simulink model "ScriptDemo"  (R2022b)
settings: configuration reference "TmVcThermal_Configuration_sub" (kept outside this file)
undefined symbols (not defined in the file): aaaa, bbbb, cTmComprCtrl_D_u8HvacFlowTable_db, cTmComprCtrl_D_u8HvacFlowTable_sw, cTmComprCtrl_n_i16ChillCmpIMax, cTmComprCtrl_n_i16ChillCmpIMin, cTmComprCtrl_n_i16ChillCmpIMin666, cTmComprCtrl_n_i16ChillCmpPMax, cTmComprCtrl_n_i16ChillCmpPMin, cTmComprCtrl_n_i16CmpChillCoolRpmKiMax, cTmComprCtrl_n_i16CmpChillCoolRpmKiMin, cTmComprCtrl_n_i16CmpChillCoolRpmKpMax, cTmComprCtrl_n_i16CmpChillCoolRpmKpMin, cTmComprCtrl_n_i16CmpCoolRpmKiMax, cTmComprCtrl_n_i16CmpCoolRpmKiMin, cTmComprCtrl_n_i16CmpCoolRpmKpMax, cTmComprCtrl_n_i16CmpCoolRpmKpMin, cTmComprCtrl_n_i16SM4CmpHeatKiMax, cTmComprCtrl_n_i16SM4CmpHeatKiMin, cTmComprCtrl_n_i16SM4CmpHeatKpMax, cTmComprCtrl_n_i16SM4CmpHeatKpMin, cTmComprCtrl_n_i16SM5CmpHeatKiMax, cTmComprCtrl_n_i16SM5CmpHeatKiMin, cTmComprCtrl_n_i16SM5CmpHeatKpMax, cTmComprCtrl_n_i16SM5CmpHeatKpMin, cTmComprCtrl_n_i16SM6CmpHeatKiMax, cTmComprCtrl_n_i16SM6CmpHeatKiMin, cTmComprCtrl_n_i16SM6CmpHeatKpMax, cTmComprCtrl_n_i16SM6CmpHeatKpMin, cTmComprCtrl_n_u16CmpMaxSpdFanFltLimt, cTmComprCtrl_n_u16CmpMaxSpdLoSidePFltLimt, cTmComprCtrl_n_u16CmpMaxSpdSensorFltLimt, cTmComprCtrl_n_u16CompMinRpm, cTmComprCtrl_n_u16CompRpmIncThres, cTmComprCtrl_t_u16BattCooltFFPeriod, cTmComprCtrl_t_u16BattCooltPIPeriod, cTmComprCtrl_t_u16CmpCoolFFPeriod, cTmComprCtrl_t_u16CmpCoolPIPeriod, cTmComprCtrl_t_u16CoolCmpChillFFPeriod, cTmComprCtrl_t_u16CoolCmpChillPIPeriod, cTmComprCtrl_t_u16SM4CmpHeatFFPeriod, cTmComprCtrl_t_u16SM4CmpHeatPIPeriod, cTmComprCtrl_t_u16SM5CmpHeatFFPeriod, cTmComprCtrl_t_u16SM5CmpHeatPIPeriod, cTmComprCtrl_t_u16SM6CmpHeatFFPeriod, cTmComprCtrl_t_u16SM6CmpHeatPIPeriod, cTmComprCtrl_Te_EvapClearInteg, cTmComprCtrl_Te_i16HpReqTempSaturoffset, cTmComprCtrl_Te_i16SatLpReplaceDiff, cTmComprCtrl_Te_i16SM3BatDiffStartEvapDecOffset, cTmComprCtrl_Te_i16SM3EvapLo, cTmComprCtrl_Te_i16SM3TBatDiffEntEvapDecOffset, cTmComprCtrl_Te_i16SM3TBatDiffEntEvapDecOffsetQuit, cTmComprCtrl_Te_s32ErrCmpChillPIContinueCoolH, cTmComprCtrl_Te_s32ErrCmpChillPIContinueCoolL, cTmComprCtrl_Te_s32ErrCmpPIContinueChillH, cTmComprCtrl_Te_s32ErrCmpPIContinueChillL, cTmComprCtrl_Te_s32ErrCmpPIContinueCoolH, cTmComprCtrl_Te_s32ErrCmpPIContinueCoolL, cTmComprCtrl_Te_s32ErrCmpPIContinueHeatH ... (+398)
libraries: simulink x782, PCMULib x640, simulink_need_slupdate x4
(part 21 of 41)

== system ScriptDemo/Create/createMerge/After/SM4/ID26297_SM4FF ==
  sTmComprCtrl_D_u8HvacFlowLevel : Inport  OutDataTypeStr=uint8
  sTmSigProces_Te_s32TempInlet : Inport  Port=2
  sTmSigProces_Te_s32HeatrAirTReqRamp : Inport  Port=3
  sTmSigProces_Te_s32TAmb : Inport  Port=4  OutDataTypeStr=single
  Enable : EnablePort
  1-D Lookup Table : Lookup_n-D  NumberOfTableDimensions=1  BreakpointsForDimension1=tTmComprCtrl_fac_s32FFSM4CompHeatAmbFactor_X  BreakpointsForDimension1DataTypeStr=Inherit: Inherit from 'Breakpoint data'  Table=tTmComprCtrl_fac_s32FFSM4CompHeatAmbFactor  TableDataTypeStr=Inherit: Inherit from 'Table data'  ExtrapMethod=Clip  InternalRulePriority=Speed  OutDataTypeStr=Inherit: Inherit via back propagation  RndMeth=Simplest  InputSameDT=off
  Flow2Rpm : Subsystem  mask{BlwHeatLevel_db=cTmComprCtrl_D_u8HvacFlowTable_db, BlwHeatLevel_sw=cTmComprCtrl_D_u8HvacFlowTable_sw, FFBlw1=mTmComprCtrl_n_u16FFSM4CompHeatRpm_Flow1, FFBlw1_Y=mTmComprCtrl_n_u16FFSM4CompHeatRpm_Flow1_Y, FFBlw1_X=mTmComprCtrl_n_u16FFSM4CompHeatRpm_Flow1_X, FFBlw3=mTmComprCtrl_n_u16FFSM4CompHeatRpm_Flow3, FFBlw3_Y=mTmComprCtrl_n_u16FFSM4CompHeatRpm_Flow3_Y, FFBlw3_X=mTmComprCtrl_n_u16FFSM4CompHeatRpm_Flow3_X, FFBlw5=mTmComprCtrl_n_u16FFSM4CompHeatRpm_Flow5, FFBlw5_Y=mTmComprCtrl_n_u16FFSM4CompHeatRpm_Flow5_Y, FFBlw5_X=mTmComprCtrl_n_u16FFSM4CompHeatRpm_Flow5_X, FFBlw7=mTmComprCtrl_n_u16FFSM4CompHeatRpm_Flow7, FFBlw7_Y=mTmComprCtrl_n_u16FFSM4CompHeatRpm_Flow7_Y, FFBlw7_X=mTmComprCtrl_n_u16FFSM4CompHeatRpm_Flow7_X, FFBlw9=mTmComprCtrl_n_u16FFSM4CompHeatRpm_Flow9, FFBlw9_Y=mTmComprCtrl_n_u16FFSM4CompHeatRpm_Flow9_Y, FFBlw9_X=mTmComprCtrl_n_u16FFSM4CompHeatRpm_Flow9_X}
      mask DialogControl ParameterGroupVar Prompt: 参数
  Product : Product  OutDataTypeStr=uint16
  SM4FF : Outport
  wires:
  sTmComprCtrl_D_u8HvacFlowLevel/1 -> Flow2Rpm/1(md_u8Blw)
  sTmSigProces_Te_s32TempInlet/1 -> Flow2Rpm/2(breakpoint1)
  sTmSigProces_Te_s32HeatrAirTReqRamp/1 -> Flow2Rpm/3(breakpoint2)
  [sTmSigProces_Te_s32TAmb] -> 1-D Lookup Table/1
  1-D Lookup Table/1 -> Product/2  "rTmComprCtrl_fac_s32FFSM4CompHeatAmbFactor"
  Flow2Rpm/1(Flow2Rpm) -> Product/1  "rTmComprCtrl_n_u16FFSM4CompHeatRpm"
  Product/1 -> SM4FF/1
  sTmSigProces_Te_s32TAmb/1 -> [sTmSigProces_Te_s32TAmb]

== system ScriptDemo/Create/createMerge/After/SM4/SM24FFEnable ==
  xTmComprCtrl_B_CompOnReqCompOn : Inport  OutDataTypeStr=boolean
  Compare To Constant2 : simulink/Logic and Bit Operations/Compare To Constant  relop===  const=0  OutDataTypeStr=boolean
  Compare To Constant3 : simulink/Logic and Bit Operations/Compare To Constant  relop===  const=1  OutDataTypeStr=boolean
  Logical Operator3 : Logic  AllPortsSameDT=off  OutDataTypeStr=boolean
  PeriodTrig : Subsystem  mask{CounterLim=cTmComprCtrl_t_u16SM4CmpHeatFFPeriod}
      mask DialogControl ParameterGroupVar Prompt: 参数
  Unit Delay : UnitDelay  SampleTime=-1  HasFrameUpgradeWarning=on
  SM4FFEnable_B_SM4FFEnable : Outport  OutDataTypeStr=boolean
  wires:
  Unit Delay/1 -> Compare To Constant2/1
  [xTmComprCtrl_B_CompOnReqCompOn] -> Compare To Constant3/1, Unit Delay/1
  Compare To Constant2/1 -> Logical Operator3/1
  Logical Operator3/1 -> PeriodTrig/1(Counter_Reset)
  Compare To Constant3/1 -> Logical Operator3/2
  xTmComprCtrl_B_CompOnReqCompOn/1 -> [xTmComprCtrl_B_CompOnReqCompOn]
  PeriodTrig/1(Counter_Trig) -> SM4FFEnable_B_SM4FFEnable/1

== system ScriptDemo/Create/createMerge/After/SM4/SM4_Ki ==
  sTmComprCtrl_D_u8HvacFlowLevel : Inport  OutDataTypeStr=uint8
  sTmSigProces_Te_s32TAmb : Inport  Port=2
  rTmComprCtrl_Te_s32TempError : Inport  Port=3
  Flow2Rpm : Subsystem  mask{BlwHeatLevel_db=cTmComprCtrl_D_u8HvacFlowTable_db, BlwHeatLevel_sw=cTmComprCtrl_D_u8HvacFlowTable_sw, FFBlw1=mTmComprCtrl_n_u16KiSM4CompHeatRpm_Flow1, FFBlw1_Y=mTmComprCtrl_n_u16KiSM4CompHeatRpm_Flow1_Y, FFBlw1_X=mTmComprCtrl_n_u16KiSM4CompHeatRpm_Flow1_X, FFBlw3=mTmComprCtrl_n_u16KiSM4CompHeatRpm_Flow3, FFBlw3_Y=mTmComprCtrl_n_u16KiSM4CompHeatRpm_Flow3_Y, FFBlw3_X=mTmComprCtrl_n_u16KiSM4CompHeatRpm_Flow3_X, FFBlw5=mTmComprCtrl_n_u16KiSM4CompHeatRpm_Flow5, FFBlw5_Y=mTmComprCtrl_n_u16KiSM4CompHeatRpm_Flow5_Y, FFBlw5_X=mTmComprCtrl_n_u16KiSM4CompHeatRpm_Flow5_X, FFBlw7=mTmComprCtrl_n_u16KiSM4CompHeatRpm_Flow7, FFBlw7_Y=mTmComprCtrl_n_u16KiSM4CompHeatRpm_Flow7_Y, FFBlw7_X=mTmComprCtrl_n_u16KiSM4CompHeatRpm_Flow7_X, FFBlw9=mTmComprCtrl_n_u16KiSM4CompHeatRpm_Flow9, FFBlw9_Y=mTmComprCtrl_n_u16KiSM4CompHeatRpm_Flow9_Y, FFBlw9_X=mTmComprCtrl_n_u16KiSM4CompHeatRpm_Flow9_X}
      mask DialogControl ParameterGroupVar Prompt: 参数
  SM4Ki : Outport
  wires:
  Flow2Rpm/1(Flow2Rpm) -> SM4Ki/1  "mask"
  sTmComprCtrl_D_u8HvacFlowLevel/1 -> Flow2Rpm/1(md_u8Blw)
  sTmSigProces_Te_s32TAmb/1 -> Flow2Rpm/2(breakpoint1)
  rTmComprCtrl_Te_s32TempError/1 -> Flow2Rpm/3(breakpoint2)

== system ScriptDemo/Create/createMerge/After/SM4/SM4_Kp ==
  sTmComprCtrl_D_u8HvacFlowLevel : Inport  OutDataTypeStr=uint8
  sTmSigProces_Te_s32TAmb : Inport  Port=2
  rTmComprCtrl_Te_s32TempError : Inport  Port=3
  Flow2Rpm : Subsystem  mask{BlwHeatLevel_db=cTmComprCtrl_D_u8HvacFlowTable_db, BlwHeatLevel_sw=cTmComprCtrl_D_u8HvacFlowTable_sw, FFBlw1=mTmComprCtrl_n_u16KpSM4CompHeatRpm_Flow1, FFBlw1_Y=mTmComprCtrl_n_u16KpSM4CompHeatRpm_Flow1_Y, FFBlw1_X=mTmComprCtrl_n_u16KpSM4CompHeatRpm_Flow1_X, FFBlw3=mTmComprCtrl_n_u16KpSM4CompHeatRpm_Flow3, FFBlw3_Y=mTmComprCtrl_n_u16KpSM4CompHeatRpm_Flow3_Y, FFBlw3_X=mTmComprCtrl_n_u16KpSM4CompHeatRpm_Flow3_X, FFBlw5=mTmComprCtrl_n_u16KpSM4CompHeatRpm_Flow5, FFBlw5_Y=mTmComprCtrl_n_u16KpSM4CompHeatRpm_Flow5_Y, FFBlw5_X=mTmComprCtrl_n_u16KpSM4CompHeatRpm_Flow5_X, FFBlw7=mTmComprCtrl_n_u16KpSM4CompHeatRpm_Flow7, FFBlw7_Y=mTmComprCtrl_n_u16KpSM4CompHeatRpm_Flow7_Y, FFBlw7_X=mTmComprCtrl_n_u16KpSM4CompHeatRpm_Flow7_X, FFBlw9=mTmComprCtrl_n_u16KpSM4CompHeatRpm_Flow9, FFBlw9_Y=mTmComprCtrl_n_u16KpSM4CompHeatRpm_Flow9_Y, FFBlw9_X=mTmComprCtrl_n_u16KpSM4CompHeatRpm_Flow9_X}
      mask DialogControl ParameterGroupVar Prompt: 参数
  SM4Kp : Outport
  wires:
  Flow2Rpm/1(Flow2Rpm) -> SM4Kp/1  "mask"
  sTmComprCtrl_D_u8HvacFlowLevel/1 -> Flow2Rpm/1(md_u8Blw)
  sTmSigProces_Te_s32TAmb/1 -> Flow2Rpm/2(breakpoint1)
  rTmComprCtrl_Te_s32TempError/1 -> Flow2Rpm/3(breakpoint2)

== system ScriptDemo/Create/createMerge/After/SM5/ID26291_SM5FF ==
  note: SM5前馈值
  note: SM5前馈值修正系数
  sTmComprCtrl_D_u8HvacFlowLevel : Inport  OutDataTypeStr=uint8
  sTmSigProces_Te_s32TempInlet : Inport  Port=2
  sTmSigProces_Te_s32HeatrAirTReqRamp : Inport  Port=3
  sTmSigProces_Te_s32SatLp : Inport  Port=4
  Enable : EnablePort
  2-D Lookup Table5 : Lookup_n-D  NumberOfTableDimensions=1  BreakpointsForDimension1=tTmComprCtrl_fac_s32FFSM5CompHeatBattCooltTFactor_X  BreakpointsForDimension2=mTmComprCtrl_n_u16FFSM5CompHeatRpmOffset_X  BreakpointsForDimension1DataTypeStr=Inherit: Inherit from 'Breakpoint data'  BreakpointsForDimension2DataTypeStr=Inherit: Inherit from 'Breakpoint data'  Table=tTmComprCtrl_fac_s32FFSM5CompHeatBattCooltTFactor  TableDataTypeStr=Inherit: Inherit from 'Table data'  ExtrapMethod=Clip  InternalRulePriority=Speed  OutDataTypeStr=Inherit: Inherit via back propagation  RndMeth=Simplest  InputSameDT=off
  Data Type Conversion : DataTypeConversion  OutDataTypeStr=uint16  SaturateOnIntegerOverflow=off  RndMeth=Floor
  Flow2Rpm : Subsystem  mask{BlwHeatLevel_db=cTmComprCtrl_D_u8HvacFlowTable_db, BlwHeatLevel_sw=cTmComprCtrl_D_u8HvacFlowTable_sw, FFBlw1=mTmComprCtrl_n_u16FFSM5CompHeatRpm_Flow1, FFBlw1_Y=mTmComprCtrl_n_u16FFSM5CompHeatRpm_Flow1_Y, FFBlw1_X=mTmComprCtrl_n_u16FFSM5CompHeatRpm_Flow1_X, FFBlw3=mTmComprCtrl_n_u16FFSM5CompHeatRpm_Flow3, FFBlw3_Y=mTmComprCtrl_n_u16FFSM5CompHeatRpm_Flow3_Y, FFBlw3_X=mTmComprCtrl_n_u16FFSM5CompHeatRpm_Flow3_X, FFBlw5=mTmComprCtrl_n_u16FFSM5CompHeatRpm_Flow5, FFBlw5_Y=mTmComprCtrl_n_u16FFSM5CompHeatRpm_Flow5_Y, FFBlw5_X=mTmComprCtrl_n_u16FFSM5CompHeatRpm_Flow5_X, FFBlw7=mTmComprCtrl_n_u16FFSM5CompHeatRpm_Flow7, FFBlw7_Y=mTmComprCtrl_n_u16FFSM5CompHeatRpm_Flow7_Y, FFBlw7_X=mTmComprCtrl_n_u16FFSM5CompHeatRpm_Flow7_X, FFBlw9=mTmComprCtrl_n_u16FFSM5CompHeatRpm_Flow9, FFBlw9_Y=mTmComprCtrl_n_u16FFSM5CompHeatRpm_Flow9_Y, FFBlw9_X=mTmComprCtrl_n_u16FFSM5CompHeatRpm_Flow9_X}
      mask DialogControl ParameterGroupVar Prompt: 参数
  Product : Product  OutDataTypeStr=uint16
  SM5FF : Outport
  wires:
  sTmSigProces_Te_s32SatLp/1 -> 2-D Lookup Table5/1
  2-D Lookup Table5/1 -> Product/2  "rTmComprCtrl_fac_s32FFSM5CompHeatBattCooltTFactor"
  Product/1 -> SM5FF/1
  sTmComprCtrl_D_u8HvacFlowLevel/1 -> Flow2Rpm/1(md_u8Blw)
  sTmSigProces_Te_s32TempInlet/1 -> Flow2Rpm/2(breakpoint1)
  sTmSigProces_Te_s32HeatrAirTReqRamp/1 -> Flow2Rpm/3(breakpoint2)
  Flow2Rpm/1(Flow2Rpm) -> Data Type Conversion/1
  Data Type Conversion/1 -> Product/1  "rTmComprCtrl_n_u16FFSM5CompHeatRpm"

== system ScriptDemo/Create/createMerge/After/SM5/ID26293_SM5Error ==
  note: 未实现
      | 暖风芯体背风温度目标值∈[30, 60] ℃ 。
  note: 无PTC补热
  note: PTC 补热模式
  sTmSigProces_Te_s32SatHp : Inport
  yTmHvchCtrl_B_HpcPtcEnad : Inport  Port=2
  sTmSigProces_Te_s32HeatrAirTReqRamp : Inport  Port=3
  sTmSigProces_Te_s32HvacHexAirTFilter : Inport  Port=4
  Add2 : Sum
  Constant5 : Constant  Value=cTmComprCtrl_Te_i16HpReqTempSaturoffset
  NegAndPosCheck 4 : Subsystem  AncestorBlock=CustomLib/TempNegAndPosCheck
  NegAndPosCheck 5 : Subsystem  AncestorBlock=CustomLib/TempNegAndPosCheck
  Saturation3 : Saturate  UpperLimit=70  LowerLimit=15
  Switch2 : Switch  Criteria=u2 ~= 0  SaturateOnIntegerOverflow=off  InputSameDT=off
  Terminator : Terminator
  Terminator1 : Terminator
  Unary Minus : UnaryMinus
  rTmComprCtrl_Te_s32TempError : Outport
  wires:
  sTmSigProces_Te_s32SatHp/1 -> NegAndPosCheck 4/2(Acture)
  NegAndPosCheck 5/1(Dvt) -> Switch2/3
  sTmSigProces_Te_s32HeatrAirTReqRamp/1 -> Saturation3/1
  Switch2/1 -> Unary Minus/1
  NegAndPosCheck 5/2(Dvt_PosFlag) -> Terminator/1
  NegAndPosCheck 4/1(Dvt) -> Switch2/1
  Constant5/1 -> Add2/1
  NegAndPosCheck 4/2(Dvt_PosFlag) -> Terminator1/1
  sTmSigProces_Te_s32HvacHexAirTFilter/1 -> NegAndPosCheck 5/2(Acture)
  yTmHvchCtrl_B_HpcPtcEnad/1 -> Switch2/2
  Saturation3/1 -> NegAndPosCheck 5/1(SetPoint), Add2/2
  Add2/1 -> NegAndPosCheck 4/1(SetPoint)
  Unary Minus/1 -> rTmComprCtrl_Te_s32TempError/1

== system ScriptDemo/Create/createMerge/After/SM5/SM5FFEnable ==
  xTmComprCtrl_B_CompOnReqCompOn : Inport  OutDataTypeStr=boolean
  Compare To Constant2 : simulink/Logic and Bit Operations/Compare To Constant  relop===  const=0  OutDataTypeStr=boolean
  Compare To Constant3 : simulink/Logic and Bit Operations/Compare To Constant  relop===  const=1  OutDataTypeStr=boolean
  Logical Operator3 : Logic  AllPortsSameDT=off  OutDataTypeStr=boolean
  PeriodTrig : Subsystem  mask{CounterLim=cTmComprCtrl_t_u16SM5CmpHeatFFPeriod}
      mask DialogControl ParameterGroupVar Prompt: 参数
  Unit Delay : UnitDelay  SampleTime=-1  HasFrameUpgradeWarning=on
  SM5FFEnable_B_SM5FFEnable : Outport  OutDataTypeStr=boolean
  wires:
  Unit Delay/1 -> Compare To Constant2/1
  [xTmComprCtrl_B_CompOnReqCompOn] -> Compare To Constant3/1, Unit Delay/1
  Compare To Constant2/1 -> Logical Operator3/1
  Logical Operator3/1 -> PeriodTrig/1(Counter_Reset)
  Compare To Constant3/1 -> Logical Operator3/2
  xTmComprCtrl_B_CompOnReqCompOn/1 -> [xTmComprCtrl_B_CompOnReqCompOn]
  PeriodTrig/1(Counter_Trig) -> SM5FFEnable_B_SM5FFEnable/1

== system ScriptDemo/Create/createMerge/After/SM5/SM5_Ki ==
  sTmComprCtrl_D_u8HvacFlowLevel : Inport  OutDataTypeStr=uint8
  sTmSigProces_Te_s32SatLp : Inport  Port=2
  rTmComprCtrl_Te_s32TempError : Inport  Port=3
  Data Type Conversion : DataTypeConversion  OutDataTypeStr=uint16  SaturateOnIntegerOverflow=off  RndMeth=Floor
  Flow2Rpm : Subsystem  mask{BlwHeatLevel_db=cTmComprCtrl_D_u8HvacFlowTable_db, BlwHeatLevel_sw=cTmComprCtrl_D_u8HvacFlowTable_sw, FFBlw1=mTmComprCtrl_n_u16KiSM5CompHeatRpm_Flow1, FFBlw1_Y=mTmComprCtrl_n_u16KiSM5CompHeatRpm_Flow1_Y, FFBlw1_X=mTmComprCtrl_n_u16KiSM5CompHeatRpm_Flow1_X, FFBlw3=mTmComprCtrl_n_u16KiSM5CompHeatRpm_Flow3, FFBlw3_Y=mTmComprCtrl_n_u16KiSM5CompHeatRpm_Flow3_Y, FFBlw3_X=mTmComprCtrl_n_u16KiSM5CompHeatRpm_Flow3_X, FFBlw5=mTmComprCtrl_n_u16KiSM5CompHeatRpm_Flow5, FFBlw5_Y=mTmComprCtrl_n_u16KiSM5CompHeatRpm_Flow5_Y, FFBlw5_X=mTmComprCtrl_n_u16KiSM5CompHeatRpm_Flow5_X, FFBlw7=mTmComprCtrl_n_u16KiSM5CompHeatRpm_Flow7, FFBlw7_Y=mTmComprCtrl_n_u16KiSM5CompHeatRpm_Flow7_Y, FFBlw7_X=mTmComprCtrl_n_u16KiSM5CompHeatRpm_Flow7_X, FFBlw9=mTmComprCtrl_n_u16KiSM5CompHeatRpm_Flow9, FFBlw9_Y=mTmComprCtrl_n_u16KiSM5CompHeatRpm_Flow9_Y, FFBlw9_X=mTmComprCtrl_n_u16KiSM5CompHeatRpm_Flow9_X}
      mask DialogControl ParameterGroupVar Prompt: 参数
  SM5Ki : Outport
  wires:
  Flow2Rpm/1(Flow2Rpm) -> Data Type Conversion/1
  Data Type Conversion/1 -> SM5Ki/1
  sTmComprCtrl_D_u8HvacFlowLevel/1 -> Flow2Rpm/1(md_u8Blw)
  sTmSigProces_Te_s32SatLp/1 -> Flow2Rpm/2(breakpoint1)
  rTmComprCtrl_Te_s32TempError/1 -> Flow2Rpm/3(breakpoint2)

== system ScriptDemo/Create/createMerge/After/SM5/SM5_Kp ==
  sTmComprCtrl_D_u8HvacFlowLevel : Inport  OutDataTypeStr=uint8
  sTmSigProces_Te_s32SatLp : Inport  Port=2
  rTmComprCtrl_Te_s32TempError : Inport  Port=3
  Data Type Conversion : DataTypeConversion  OutDataTypeStr=uint16  SaturateOnIntegerOverflow=off  RndMeth=Floor
  Flow2Rpm : Subsystem  mask{BlwHeatLevel_db=cTmComprCtrl_D_u8HvacFlowTable_db, BlwHeatLevel_sw=cTmComprCtrl_D_u8HvacFlowTable_sw, FFBlw1=mTmComprCtrl_n_u16KpSM5CompHeatRpm_Flow1, FFBlw1_Y=mTmComprCtrl_n_u16KpSM5CompHeatRpm_Flow1_Y, FFBlw1_X=mTmComprCtrl_n_u16KpSM5CompHeatRpm_Flow1_X, FFBlw3=mTmComprCtrl_n_u16KpSM5CompHeatRpm_Flow3, FFBlw3_Y=mTmComprCtrl_n_u16KpSM5CompHeatRpm_Flow3_Y, FFBlw3_X=mTmComprCtrl_n_u16KpSM5CompHeatRpm_Flow3_X, FFBlw5=mTmComprCtrl_n_u16KpSM5CompHeatRpm_Flow5, FFBlw5_Y=mTmComprCtrl_n_u16KpSM5CompHeatRpm_Flow5_Y, FFBlw5_X=mTmComprCtrl_n_u16KpSM5CompHeatRpm_Flow5_X, FFBlw7=mTmComprCtrl_n_u16KpSM5CompHeatRpm_Flow7, FFBlw7_Y=mTmComprCtrl_n_u16KpSM5CompHeatRpm_Flow7_Y, FFBlw7_X=mTmComprCtrl_n_u16KpSM5CompHeatRpm_Flow7_X, FFBlw9=mTmComprCtrl_n_u16KpSM5CompHeatRpm_Flow9, FFBlw9_Y=mTmComprCtrl_n_u16KpSM5CompHeatRpm_Flow9_Y, FFBlw9_X=mTmComprCtrl_n_u16KpSM5CompHeatRpm_Flow9_X}
      mask DialogControl ParameterGroupVar Prompt: 参数
  SM5Kp : Outport
  wires:
  Flow2Rpm/1(Flow2Rpm) -> Data Type Conversion/1
  Data Type Conversion/1 -> SM5Kp/1
  sTmSigProces_Te_s32SatLp/1 -> Flow2Rpm/2(breakpoint1)
  rTmComprCtrl_Te_s32TempError/1 -> Flow2Rpm/3(breakpoint2)
  sTmComprCtrl_D_u8HvacFlowLevel/1 -> Flow2Rpm/1(md_u8Blw)

== system ScriptDemo/Create/createMerge/After/SM6/ID26282_SM6FF ==
  note: TODO: 这里需要确认下需求
  sTmComprCtrl_D_u8HvacFlowLevel : Inport  OutDataTypeStr=uint8
  sTmSigProces_Te_s32TempInlet : Inport  Port=2
  sTmSigProces_Te_s32HeatrAirTReqRamp : Inport  Port=3
  Enable : EnablePort
  Flow2Rpm : Subsystem  mask{BlwHeatLevel_db=cTmComprCtrl_D_u8HvacFlowTable_db, BlwHeatLevel_sw=cTmComprCtrl_D_u8HvacFlowTable_sw, FFBlw1=mTmComprCtrl_n_u16FFSM6CompHeatRpm_Flow1, FFBlw1_Y=mTmComprCtrl_n_u16FFSM6CompHeatRpm_Flow1_Y, FFBlw1_X=mTmComprCtrl_n_u16FFSM6CompHeatRpm_Flow1_X, FFBlw3=mTmComprCtrl_n_u16FFSM6CompHeatRpm_Flow3, FFBlw3_Y=mTmComprCtrl_n_u16FFSM6CompHeatRpm_Flow3_Y, FFBlw3_X=mTmComprCtrl_n_u16FFSM6CompHeatRpm_Flow3_X, FFBlw5=mTmComprCtrl_n_u16FFSM6CompHeatRpm_Flow5, FFBlw5_Y=mTmComprCtrl_n_u16FFSM6CompHeatRpm_Flow5_Y, FFBlw5_X=mTmComprCtrl_n_u16FFSM6CompHeatRpm_Flow5_X, FFBlw7=mTmComprCtrl_n_u16FFSM6CompHeatRpm_Flow7, FFBlw7_Y=mTmComprCtrl_n_u16FFSM6CompHeatRpm_Flow7_Y, FFBlw7_X=mTmComprCtrl_n_u16FFSM6CompHeatRpm_Flow7_X, FFBlw9=mTmComprCtrl_n_u16FFSM6CompHeatRpm_Flow9, FFBlw9_Y=mTmComprCtrl_n_u16FFSM6CompHeatRpm_Flow9_Y, FFBlw9_X=mTmComprCtrl_n_u16FFSM6CompHeatRpm_Flow9_X}
      mask DialogControl ParameterGroupVar Prompt: 参数
  SM6FF : Outport
  wires:
  Flow2Rpm/1(Flow2Rpm) -> SM6FF/1
  sTmComprCtrl_D_u8HvacFlowLevel/1 -> Flow2Rpm/1(md_u8Blw)
  sTmSigProces_Te_s32HeatrAirTReqRamp/1 -> Flow2Rpm/3(breakpoint2)
  sTmSigProces_Te_s32TempInlet/1 -> Flow2Rpm/2(breakpoint1)

== system ScriptDemo/Create/createMerge/After/SM6/ID26284_SM6Error ==
  note: 暖风芯体背风温度目标值∈[0, 80] ℃ 。
  note: 无PTC补热
  note: PTC 补热模式
  sTmSigProces_Te_s32SatHp : Inport
  yTmHvchCtrl_B_HpcPtcEnad : Inport  Port=2
  sTmSigProces_Te_s32HeatrAirTReqRamp : Inport  Port=3
  sTmSigProces_Te_s32HvacHexAirTFilter : Inport  Port=4
  Add2 : Sum
  Constant5 : Constant  Value=cTmComprCtrl_Te_i16HpReqTempSaturoffset
  NegAndPosCheck 4 : Subsystem  AncestorBlock=CustomLib/TempNegAndPosCheck
  NegAndPosCheck 5 : Subsystem  AncestorBlock=CustomLib/TempNegAndPosCheck
  Saturation2 : Saturate  UpperLimit=70  LowerLimit=15
  Switch2 : Switch  Criteria=u2 ~= 0  SaturateOnIntegerOverflow=off  InputSameDT=off
  Terminator : Terminator
  Terminator1 : Terminator
  Unary Minus : UnaryMinus
  rTmComprCtrl_Te_s32TempError : Outport
  wires:
  sTmSigProces_Te_s32SatHp/1 -> NegAndPosCheck 4/2(Acture)
  NegAndPosCheck 5/1(Dvt) -> Switch2/3
  sTmSigProces_Te_s32HeatrAirTReqRamp/1 -> Saturation2/1
  Switch2/1 -> Unary Minus/1
  NegAndPosCheck 5/2(Dvt_PosFlag) -> Terminator/1
  NegAndPosCheck 4/1(Dvt) -> Switch2/1
  Constant5/1 -> Add2/1
  NegAndPosCheck 4/2(Dvt_PosFlag) -> Terminator1/1
  sTmSigProces_Te_s32HvacHexAirTFilter/1 -> NegAndPosCheck 5/2(Acture)
  yTmHvchCtrl_B_HpcPtcEnad/1 -> Switch2/2
  Saturation2/1 -> NegAndPosCheck 5/1(SetPoint), Add2/2
  Add2/1 -> NegAndPosCheck 4/1(SetPoint)
  Unary Minus/1 -> rTmComprCtrl_Te_s32TempError/1

== system ScriptDemo/Create/createMerge/After/SM6/SM6FFEnable ==
  xTmComprCtrl_B_CompOnReqCompOn : Inport  OutDataTypeStr=boolean
  Compare To Constant2 : simulink/Logic and Bit Operations/Compare To Constant  relop===  const=0  OutDataTypeStr=boolean
  Compare To Constant3 : simulink/Logic and Bit Operations/Compare To Constant  relop===  const=1  OutDataTypeStr=boolean
  Logical Operator3 : Logic  AllPortsSameDT=off  OutDataTypeStr=boolean
  PeriodTrig : Subsystem  mask{CounterLim=cTmComprCtrl_t_u16SM6CmpHeatFFPeriod}
      mask DialogControl ParameterGroupVar Prompt: 参数
  Unit Delay : UnitDelay  SampleTime=-1  HasFrameUpgradeWarning=on
  SM6FFEnable_B_SM6FFEnable : Outport  OutDataTypeStr=boolean
  wires:
  Unit Delay/1 -> Compare To Constant2/1
  [xTmComprCtrl_B_CompOnReqCompOn] -> Compare To Constant3/1, Unit Delay/1
  Compare To Constant2/1 -> Logical Operator3/1
  Logical Operator3/1 -> PeriodTrig/1(Counter_Reset)
  Compare To Constant3/1 -> Logical Operator3/2
  xTmComprCtrl_B_CompOnReqCompOn/1 -> [xTmComprCtrl_B_CompOnReqCompOn]
  PeriodTrig/1(Counter_Trig) -> SM6FFEnable_B_SM6FFEnable/1

== system ScriptDemo/Create/createMerge/After/SM6/SM6_Ki ==
  sTmComprCtrl_D_u8HvacFlowLevel : Inport  OutDataTypeStr=uint8
  sTmSigProces_Te_s32TempInlet : Inport  Port=2
  rTmComprCtrl_Te_s32TempError : Inport  Port=3
  Flow2Rpm : Subsystem  mask{BlwHeatLevel_db=cTmComprCtrl_D_u8HvacFlowTable_db, BlwHeatLevel_sw=cTmComprCtrl_D_u8HvacFlowTable_sw, FFBlw1=mTmComprCtrl_n_u16KiSM6CompHeatRpm_Flow1, FFBlw1_Y=mTmComprCtrl_n_u16KiSM6CompHeatRpm_Flow1_Y, FFBlw1_X=mTmComprCtrl_n_u16KiSM6CompHeatRpm_Flow1_X, FFBlw3=mTmComprCtrl_n_u16KiSM6CompHeatRpm_Flow3, FFBlw3_Y=mTmComprCtrl_n_u16KiSM6CompHeatRpm_Flow3_Y, FFBlw3_X=mTmComprCtrl_n_u16KiSM6CompHeatRpm_Flow3_X, FFBlw5=mTmComprCtrl_n_u16KiSM6CompHeatRpm_Flow5, FFBlw5_Y=mTmComprCtrl_n_u16KiSM6CompHeatRpm_Flow5_Y, FFBlw5_X=mTmComprCtrl_n_u16KiSM6CompHeatRpm_Flow5_X, FFBlw7=mTmComprCtrl_n_u16KiSM6CompHeatRpm_Flow7, FFBlw7_Y=mTmComprCtrl_n_u16KiSM6CompHeatRpm_Flow7_Y, FFBlw7_X=mTmComprCtrl_n_u16KiSM6CompHeatRpm_Flow7_X, FFBlw9=mTmComprCtrl_n_u16KiSM6CompHeatRpm_Flow9, FFBlw9_Y=mTmComprCtrl_n_u16KiSM6CompHeatRpm_Flow9_Y, FFBlw9_X=mTmComprCtrl_n_u16KiSM6CompHeatRpm_Flow9_X}
      mask DialogControl ParameterGroupVar Prompt: 参数
  SM6Ki : Outport
  wires:
  Flow2Rpm/1(Flow2Rpm) -> SM6Ki/1
  sTmSigProces_Te_s32TempInlet/1 -> Flow2Rpm/2(breakpoint1)
  sTmComprCtrl_D_u8HvacFlowLevel/1 -> Flow2Rpm/1(md_u8Blw)
  rTmComprCtrl_Te_s32TempError/1 -> Flow2Rpm/3(breakpoint2)

== system ScriptDemo/Create/createMerge/After/SM6/SM6_Kp ==
  sTmComprCtrl_D_u8HvacFlowLevel : Inport  OutDataTypeStr=uint8
  sTmSigProces_Te_s32TempInlet : Inport  Port=2
  rTmComprCtrl_Te_s32TempError : Inport  Port=3
  Flow2Rpm : Subsystem  mask{BlwHeatLevel_db=cTmComprCtrl_D_u8HvacFlowTable_db, BlwHeatLevel_sw=cTmComprCtrl_D_u8HvacFlowTable_sw, FFBlw1=mTmComprCtrl_n_u16KpSM6CompHeatRpm_Flow1, FFBlw1_Y=mTmComprCtrl_n_u16KpSM6CompHeatRpm_Flow1_Y, FFBlw1_X=mTmComprCtrl_n_u16KpSM6CompHeatRpm_Flow1_X, FFBlw3=mTmComprCtrl_n_u16KpSM6CompHeatRpm_Flow3, FFBlw3_Y=mTmComprCtrl_n_u16KpSM6CompHeatRpm_Flow3_Y, FFBlw3_X=mTmComprCtrl_n_u16KpSM6CompHeatRpm_Flow3_X, FFBlw5=mTmComprCtrl_n_u16KpSM6CompHeatRpm_Flow5, FFBlw5_Y=mTmComprCtrl_n_u16KpSM6CompHeatRpm_Flow5_Y, FFBlw5_X=mTmComprCtrl_n_u16KpSM6CompHeatRpm_Flow5_X, FFBlw7=mTmComprCtrl_n_u16KpSM6CompHeatRpm_Flow7, FFBlw7_Y=mTmComprCtrl_n_u16KpSM6CompHeatRpm_Flow7_Y, FFBlw7_X=mTmComprCtrl_n_u16KpSM6CompHeatRpm_Flow7_X, FFBlw9=mTmComprCtrl_n_u16KpSM6CompHeatRpm_Flow9, FFBlw9_Y=mTmComprCtrl_n_u16KpSM6CompHeatRpm_Flow9_Y, FFBlw9_X=mTmComprCtrl_n_u16KpSM6CompHeatRpm_Flow9_X}
      mask DialogControl ParameterGroupVar Prompt: 参数
  SM6Kp : Outport
  wires:
  Flow2Rpm/1(Flow2Rpm) -> SM6Kp/1
  sTmComprCtrl_D_u8HvacFlowLevel/1 -> Flow2Rpm/1(md_u8Blw)
  sTmSigProces_Te_s32TempInlet/1 -> Flow2Rpm/2(breakpoint1)
  rTmComprCtrl_Te_s32TempError/1 -> Flow2Rpm/3(breakpoint2)

== system ScriptDemo/Create/createMerge/Before/ID29332_RpmPI/ClearInteg ==
  rPIControler_n_s32SAccmKi : Inport  OutDataTypeStr=single
  sTmRefriModeMgr_D_u8HPCurMode : Inport  Port=2  OutDataTypeStr=uint8
  sTmSigProces_Te_s32EvapFanFilter : Inport  Port=3  OutDataTypeStr=single
  xTmComprCtrl_B_CompOnReqCompOn : Inport  Port=4  OutDataTypeStr=boolean
  xTmComprCtrl_B_ModeChanged : Inport  Port=5  OutDataTypeStr=boolean
  yTmRefriModeMgr_B_CoolModeInCycle : Inport  Port=6  OutDataTypeStr=boolean
  yTmRefriModeMgr_B_HeatModeInCycle : Inport  Port=7  OutDataTypeStr=boolean
  Compare To Constant : simulink/Logic and Bit Operations/Compare To Constant  relop===  const=0  OutDataTypeStr=boolean
  Compare To Constant1 : simulink/Logic and Bit Operations/Compare To Constant  relop=>  const=0  OutDataTypeStr=boolean
  Compare To Constant2 : simulink/Logic and Bit Operations/Compare To Constant  relop===  const=[2 22]  OutDataTypeStr=boolean
  Compare To Constant3 : simulink/Logic and Bit Operations/Compare To Constant  relop=<=  const=cTmComprCtrl_Te_EvapClearInteg  OutDataTypeStr=boolean
  Logical Operator : Logic  Operator=OR  Inputs=4  AllPortsSameDT=off  OutDataTypeStr=boolean
  Logical Operator1 : Logic  Inputs=3  AllPortsSameDT=off  OutDataTypeStr=boolean
  Logical Operator2 : Logic  Operator=OR  Inputs=1  AllPortsSameDT=off  OutDataTypeStr=boolean
  Logical Operator3 : Logic  Operator=OR  AllPortsSameDT=off  OutDataTypeStr=boolean
  Unit Delay : UnitDelay  SampleTime=-1  HasFrameUpgradeWarning=on
  xClearInteg_B_ClearInteg : Outport  OutDataTypeStr=boolean
  wires:
  [xTmComprCtrl_B_ModeChanged] -> Logical Operator/2
  Compare To Constant/1 -> Logical Operator/1
  [xTmComprCtrl_B_CompOnReqCompOn] -> Compare To Constant/1
  Logical Operator/1 -> [xTmComprCtrl_B_ClearInteg]  "xTmComprCtrl_B_ClearInteg"
  [rPIControler_n_s32SAccmKi] -> Unit Delay/1
  [sTmRefriModeMgr_D_u8HPCurMode] -> Compare To Constant2/1
  [sTmSigProces_Te_s32EvapFanFilter] -> Compare To Constant3/1
  Compare To Constant2/1 -> Logical Operator2/1
  Compare To Constant1/1 -> Logical Operator1/1
  Compare To Constant3/1 -> Logical Operator1/3
  Logical Operator1/1 -> Logical Operator/3
  rPIControler_n_s32SAccmKi/1 -> [rPIControler_n_s32SAccmKi]
  sTmRefriModeMgr_D_u8HPCurMode/1 -> [sTmRefriModeMgr_D_u8HPCurMode]
  sTmSigProces_Te_s32EvapFanFilter/1 -> [sTmSigProces_Te_s32EvapFanFilter]
  xTmComprCtrl_B_CompOnReqCompOn/1 -> [xTmComprCtrl_B_CompOnReqCompOn]
  xTmComprCtrl_B_ModeChanged/1 -> [xTmComprCtrl_B_ModeChanged]
  [xTmComprCtrl_B_ClearInteg] -> xClearInteg_B_ClearInteg/1
  Unit Delay/1 -> Compare To Constant1/1
  Logical Operator2/1 -> Logical Operator1/2
  [yTmRefriModeMgr_B_CoolModeInCycle] -> Logical Operator3/1
  [yTmRefriModeMgr_B_HeatModeInCycle] -> Logical Operator3/2
  Logical Operator3/1 -> Logical Operator/4
  yTmRefriModeMgr_B_CoolModeInCycle/1 -> [yTmRefriModeMgr_B_CoolModeInCycle]
  yTmRefriModeMgr_B_HeatModeInCycle/1 -> [yTmRefriModeMgr_B_HeatModeInCycle]

== system ScriptDemo/Create/createMerge/Before/ID29332_RpmPI/PIControler ==
  note: 新增观测量rTmComprCtrl_n_u16CompRpmReqPIRaw，rTmComprCtrl_n_u16CompRpmReqPI为边界限制后的PI输出
  note: 0=Not saturated
      | 1=Saturated TOP
      | 2=SaturatedBottom
      | 3=Saturated both (?!?)
  xTmComprCtrl_B_Enable : Inport  OutDataTypeStr=boolean
  xTmComprCtrl_B_ClearInteg : Inport  Port=2  OutDataTypeStr=boolean
  rTmComprCtrl_t_u16PIPeriod : Inport  Port=3  OutDataTypeStr=uint16
  rTmComprCtrl_Te_s32TempError : Inport  Port=4  OutDataTypeStr=single
  rTmComprCtrl_n_u16ComprRpmFF : Inport  Port=5  OutDataTypeStr=uint16
  rTmComprCtrl_n_u16ComprRpmKp : Inport  Port=6  OutDataTypeStr=uint16
  rTmComprCtrl_n_u16ComprRpmKi : Inport  Port=7  OutDataTypeStr=uint16
  rTmComprCtrl_n_i16KpUpLimit : Inport  Port=8  OutDataTypeStr=int16
  rTmComprCtrl_n_i16KpLowLimit : Inport  Port=9  OutDataTypeStr=int16
  rTmComprCtrl_n_i16KiUpLimit : Inport  Port=10  OutDataTypeStr=int16
  rTmComprCtrl_n_i16KiLowLimit : Inport  Port=11  OutDataTypeStr=int16
  rTmComprCtrl_Te_s32UpErrStop : Inport  Port=12  OutDataTypeStr=single
  rTmComprCtrl_Te_s32LowErrStop : Inport  Port=13  OutDataTypeStr=single
  rTmComprCtrl_n_u16DisOverrideValue : Inport  Port=14  OutDataTypeStr=uint16
  xTmComprCtrl_B_ReduceRpm : Inport  Port=15  OutDataTypeStr=boolean
  Constant : Constant  Value=0  OutDataTypeStr=single
  Constant1 : Constant  Commented=on  Value=0  OutDataTypeStr=uint16
  Constant10 : Constant  Value=8000  OutDataTypeStr=uint16
  Constant11 : Constant  Value=cTmComprCtrl_n_u16CompMinRpm  OutDataTypeStr=uint16
  Constant12 : Constant  Value=0  OutDataTypeStr=single
  Constant13 : Constant  Value=0  OutDataTypeStr=single
  Constant14 : Constant  Commented=on  Value=0  OutDataTypeStr=int16
  Constant2 : Constant  Value=cTmSwArch_t_s32SampleTime  OutDataTypeStr=single
  Constant3 : Constant  Commented=on  Value=0  OutDataTypeStr=int16
  Data Type Conversion : DataTypeConversion  OutDataTypeStr=uint16  RndMeth=Floor
  Data Type Conversion1 : DataTypeConversion  OutDataTypeStr=single  RndMeth=Floor
  Data Type Conversion4 : DataTypeConversion  OutDataTypeStr=uint16  SaturateOnIntegerOverflow=off  RndMeth=Floor
  From10 : From  Commented=on  GotoTag=rTmComprCtrl_n_i16KdLowLimit
  From17 : From  Commented=on  GotoTag=rTmComprCtrl_Te_s32TempError
  From4 : From  Commented=on  GotoTag=rTmComprCtrl_n_u16ComprRpmKd
  From9 : From  Commented=on  GotoTag=rTmComprCtrl_n_i16KdUpLimit
  Goto10 : Goto  Commented=on  GotoTag=rTmComprCtrl_n_u16ComprRpmKd
  Goto14 : Goto  Commented=on  GotoTag=rTmComprCtrl_n_i16KdLowLimit
  Goto15 : Goto  Commented=on  GotoTag=rTmComprCtrl_n_i16KdUpLimit
  Integral Multiply : Product  OutDataTypeStr=single  RndMeth=Zero  SaturateOnIntegerOverflow=on
  PID_Saturation : Subsystem  mask(Saturation Dynamic){OutMin=[], OutMax=[], OutDataTypeStr=Inherit: Same as second input, OutputDataTypeScalingMode=Same as second input, OutDataType=FloatBit1, OutScaling=[], LockScale=off, RndMeth=Nearest, DoSatur=on}
      mask prompts: OutMin "Output minimum:"; OutMax "Output maximum:"; OutDataTypeStr "Output data type:"; OutputDataTypeScalingMode "Output data type mode:"; OutDataType "Output data type (e.g. fixdt(1, 16), fixdt('single')):"; OutScaling "Output scaling (Slope, e.g. 2^-9 or [Slope Bias], e.g. [1.25 3]):"; LockScale "Lock output data type setting against changes by the fixed-point tools"; RndMeth "Integer rounding mode:"; DoSatur "Saturate on integer overflow"
      mask help: Bound the range of the second input by using the first input (upper limit) and the third input (lower limit).
      mask init: same as ScriptDemo/Create/createMerge/After/ID29332_RpmPI/PIControler/PID_Saturation
      mask Callback OutDataTypeStr: fixptdialog(gcbh)
      mask TypeOptions OutputDataTypeScalingMode: double | single | int8 | uint8 | int16 | uint16 | int32 | uint32 | Specify via dialog | Same as second input
      mask Callback OutputDataTypeScalingMode: fixptdialog(gcbh)
      mask Callback OutDataType: fixptdialog(gcbh)
      mask TypeOptions RndMeth: Ceiling | Convergent | Floor | Nearest | Round | Simplest | Zero
      mask Display: plot([0.15 0.85],[.5 .5],[.5 .5],[0.05 0.95],0.15+0.7*[0 .25 .75 1],0.05+0.9*[.25 .25 .75 .75]);
  Product : Product  OutDataTypeStr=single  RndMeth=Zero
  Product2 : Product  Commented=on  OutDataTypeStr=single  RndMeth=Zero  SaturateOnIntegerOverflow=on
  Product3 : Product  Inputs=**/  OutDataTypeStr=single
  Saturation Dynamic : simulink/Discontinuities/Saturation Dynamic  OutMin=[]  OutMax=[]  OutDataTypeStr=Inherit: Same as second input  OutDataType=fixdt(1, 16)  OutScaling=2^-10  DoSatur=off
  Saturation Dynamic1 : simulink/Discontinuities/Saturation Dynamic  OutMin=[]  OutMax=[]  OutDataTypeStr=Inherit: Same as second input  OutDataType=fixdt(1, 16)  OutScaling=2^-10  DoSatur=off
  Saturation Dynamic2 : simulink/Discontinuities/Saturation Dynamic  Commented=on  OutMin=[]  OutMax=[]  OutDataTypeStr=Inherit: Same as second input  OutDataType=fixdt(1, 16)  OutScaling=2^-10  DoSatur=off
  SaturationAndDeadband : Subsystem
  Sum1 : Sum  Inputs=|++  InputSameDT=on  AccumDataTypeStr=single  OutDataTypeStr=single  SaturateOnIntegerOverflow=on
  Sum2 : Sum  Commented=on  Inputs=|+-  SaturateOnIntegerOverflow=on
  Sum4 : Sum  Inputs=++++  OutDataTypeStr=single  RndMeth=Nearest  SaturateOnIntegerOverflow=on
  Switch : Switch  Criteria=u2 ~= 0  SaturateOnIntegerOverflow=off  InputSameDT=off
  Unit Delay : UnitDelay  Commented=on  SampleTime=-1  HasFrameUpgradeWarning=on
  Unit Delay Resettable External IC : simulink_need_slupdate/Unit Delay Resettable External IC  tsamp=-1
  Unit Delay1 : UnitDelay  SampleTime=-1  HasFrameUpgradeWarning=on
  rPIControler_n_u16CompRpmReq : Outport  OutDataTypeStr=uint16
  rPIControler_n_s32SAccmKi : Outport  Port=2  OutDataTypeStr=single
  wires:
  Constant/1 -> Sum4/3  "rTmComprCtrl_n_s32SAccmKd"
  Data Type Conversion4/1 -> [rTmComprCtrl_n_u16CompRpmReq]
  [rTmComprCtrl_n_u16ComprRpmKp] -> Product/1
  Product3/1 -> Integral Multiply/2
  Switch/1 -> Data Type Conversion4/1
  Integral Multiply/1 -> Sum1/1
  Product/1 -> Saturation Dynamic/2
  Sum4/1 -> Data Type Conversion/1
  SaturationAndDeadband/1(rSaturationAndDeadband_Te_s32TempErrorOut) -> Integral Multiply/1  "rTmComprCtrl_Te_s32TempErrorInteg"
  [rTmComprCtrl_n_u16OutLowLimit] -> PID_Saturation/3(lo)
  [rTmComprCtrl_Te_s32InitialIntegral] -> Unit Delay Resettable External IC/3  "rTmComprCtrl_Te_s32InitialIntegral"
  Unit Delay Resettable External IC/1 -> Sum1/2  "Integrator"
  From17/1 -> Unit Delay/1, Sum2/1
  Unit Delay/1 -> Sum2/2
  [rTmComprCtrl_n_u16OutUpLimit] -> PID_Saturation/1(up)
  Constant2/1 -> Product3/2
  [rTmComprCtrl_t_u16PIPeriod] -> Product3/3
  [rTmComprCtrl_n_u16ComprRpmKi] -> Product3/1
  Saturation Dynamic1/1 -> Sum4/4, [rTmComprCtrl_n_s32SAccmKi], Unit Delay Resettable External IC/1  "rTmComprCtrl_n_s32SAccmKi"
  [rTmComprCtrl_n_u16ComprRpmFF] -> Data Type Conversion1/1
  [rTmComprCtrl_n_i16KpUpLimit] -> Saturation Dynamic/1
  [rTmComprCtrl_n_i16KpLowLimit] -> Saturation Dynamic/3
  [rTmComprCtrl_Te_s32TempError] -> Product/2
  Saturation Dynamic/1 -> Sum4/2  "rTmComprCtrl_n_s32SAccmKp"
  Sum1/1 -> Saturation Dynamic1/2
  [rTmComprCtrl_n_i16KiUpLimit] -> Saturation Dynamic1/1
  [rTmComprCtrl_n_i16KiLowLimit] -> Saturation Dynamic1/3
  [rTmComprCtrl_Te_s32DeadBand] -> SaturationAndDeadband/2(rTmComprCtrl_Te_s32DeadBand)
  PID_Saturation/2(N_SaturationState) -> Unit Delay1/1
  Unit Delay1/1 -> [N_SaturationState]
  [rTmComprCtrl_n_u16DisOverrideValue] -> Switch/3
  PID_Saturation/1(y) -> [rTmComprCtrl_n_u16CompRpmPi]
  [rTmComprCtrl_n_u16CompRpmPi] -> Switch/1
  [xTmComprCtrl_B_Enable] -> Switch/2
  [N_SaturationState] -> SaturationAndDeadband/1(N_SaturationState)
  [rTmComprCtrl_Te_s32TempError] -> SaturationAndDeadband/4(rTmComprCtrl_Te_s32TempError)
  [rTmComprCtrl_Te_s32UpErrStop] -> SaturationAndDeadband/5(rTmComprCtrl_Te_s32UpErrStop)
  [rTmComprCtrl_Te_s32LowErrStop] -> SaturationAndDeadband/3(rTmComprCtrl_Te_s32LowErrStop)
  Product2/1 -> Saturation Dynamic2/2
  From10/1 -> Saturation Dynamic2/3
  From9/1 -> Saturation Dynamic2/1
  From4/1 -> Product2/1
  Sum2/1 -> Product2/2
  rTmComprCtrl_Te_s32LowErrStop/1 -> [rTmComprCtrl_Te_s32LowErrStop]
  rTmComprCtrl_Te_s32TempError/1 -> [rTmComprCtrl_Te_s32TempError]
  rTmComprCtrl_Te_s32UpErrStop/1 -> [rTmComprCtrl_Te_s32UpErrStop]
  rTmComprCtrl_n_u16ComprRpmFF/1 -> [rTmComprCtrl_n_u16ComprRpmFF]
  rTmComprCtrl_n_u16ComprRpmKi/1 -> [rTmComprCtrl_n_u16ComprRpmKi]
  rTmComprCtrl_n_u16ComprRpmKp/1 -> [rTmComprCtrl_n_u16ComprRpmKp]
  rTmComprCtrl_n_u16DisOverrideValue/1 -> [rTmComprCtrl_n_u16DisOverrideValue]
  Constant14/1 -> Goto14/1
  rTmComprCtrl_n_i16KiLowLimit/1 -> [rTmComprCtrl_n_i16KiLowLimit]
  rTmComprCtrl_n_i16KiUpLimit/1 -> [rTmComprCtrl_n_i16KiUpLimit]
  rTmComprCtrl_n_i16KpLowLimit/1 -> [rTmComprCtrl_n_i16KpLowLimit]
  Constant11/1 -> [rTmComprCtrl_n_u16OutLowLimit]
  rTmComprCtrl_t_u16PIPeriod/1 -> [rTmComprCtrl_t_u16PIPeriod]
  [rTmComprCtrl_n_u16CompRpmReq] -> rPIControler_n_u16CompRpmReq/1  "rPIControler_n_u16CompRpmReq"
  Data Type Conversion1/1 -> Sum4/1  "FF"
  Data Type Conversion/1 -> PID_Saturation/2(u)  "PI"
  xTmComprCtrl_B_ReduceRpm/1 -> [xTmComprCtrl_B_ReduceRpm]
  xTmComprCtrl_B_Enable/1 -> [xTmComprCtrl_B_Enable]
  Constant1/1 -> Goto10/1
  rTmComprCtrl_n_i16KpUpLimit/1 -> [rTmComprCtrl_n_i16KpUpLimit]
  Constant3/1 -> Goto15/1
  Constant10/1 -> [rTmComprCtrl_n_u16OutUpLimit]
  Constant12/1 -> [rTmComprCtrl_Te_s32InitialIntegral]
  xTmComprCtrl_B_ClearInteg/1 -> [xTmComprCtrl_B_ClearInteg]
  [xTmComprCtrl_B_ClearInteg] -> Unit Delay Resettable External IC/2  "xTmComprCtrl_B_ClearInteg"
  Constant13/1 -> [rTmComprCtrl_Te_s32DeadBand]
  [xTmComprCtrl_B_ReduceRpm] -> SaturationAndDeadband/6(xTmComprCtrl_B_ReduceRpm)
  [rTmComprCtrl_n_s32SAccmKi] -> rPIControler_n_s32SAccmKi/1

== system ScriptDemo/Create/createMerge/Before/SM1SM21/ID26245_SM1FF ==
  sTmIn_Te_s32HvBattCooltTReq : Inport
  sTmIn_D_u8DCChrgSt : Inport  Port=2  OutDataTypeStr=uint8
  sTmSigProces_D_u8HvBattCoolgReq : Inport  Port=3  OutDataTypeStr=uint8
  sTmSigProces_Te_s32TAmb : Inport  Port=4  OutDataTypeStr=single
  sTmIn_D_u8HeatPump : Inport  Port=5  OutDataTypeStr=uint8
  Enable : EnablePort
  1-D Lookup Table : Lookup_n-D  NumberOfTableDimensions=1  BreakpointsForDimension1=tTmComprCtrl_fac_s32SM1FFTFactor_X  BreakpointsForDimension1DataTypeStr=Inherit: Inherit from 'Breakpoint data'  Table=tTmComprCtrl_fac_s32SM1FFTFactor  TableDataTypeStr=Inherit: Inherit from 'Table data'  ExtrapMethod=Clip  InternalRulePriority=Speed  OutDataTypeStr=Inherit: Inherit via back propagation  RndMeth=Simplest  InputSameDT=off
  2-D Lookup Table : Lookup_n-D  BreakpointsForDimension1=mTmComprCtrl_n_u16FFBattCooltRpmNorm_Y  BreakpointsForDimension2=mTmComprCtrl_n_u16FFBattCooltRpmNorm_X  BreakpointsForDimension1DataTypeStr=Inherit: Inherit from 'Breakpoint data'  BreakpointsForDimension2DataTypeStr=Inherit: Inherit from 'Breakpoint data'  Table=mTmComprCtrl_n_u16FFBattCooltRpmNorm  TableDataTypeStr=Inherit: Inherit from 'Table data'  ExtrapMethod=Clip  InternalRulePriority=Speed  OutDataTypeStr=Inherit: Inherit via back propagation  RndMeth=Simplest  InputSameDT=off
      settings: InputPortMap=u0,u1
  2-D Lookup Table1 : Lookup_n-D  BreakpointsForDimension1=mTmComprCtrl_n_u16FFBattCooltRpmNormNhp_Y  BreakpointsForDimension2=mTmComprCtrl_n_u16FFBattCooltRpmNormNhp_X  BreakpointsForDimension1DataTypeStr=Inherit: Inherit from 'Breakpoint data'  BreakpointsForDimension2DataTypeStr=Inherit: Inherit from 'Breakpoint data'  Table=mTmComprCtrl_n_u16FFBattCooltRpmNormNhp  TableDataTypeStr=Inherit: Inherit from 'Table data'  ExtrapMethod=Clip  InternalRulePriority=Speed  OutDataTypeStr=Inherit: Inherit via back propagation  RndMeth=Simplest  InputSameDT=off
      settings: InputPortMap=u0,u1
  2-D Lookup Table2 : Lookup_n-D  LookupTableObject=mTmComprCtrl_n_u16FFBattCooltRpmCharging  BreakpointsForDimension1=mTmComprCtrl_n_u16FFBattCooltRpmChargingNhp_Y  BreakpointsForDimension2=mTmComprCtrl_n_u16FFBattCooltRpmChargingNhp_X  BreakpointsForDimension1DataTypeStr=Inherit: Inherit from 'Breakpoint data'  BreakpointsForDimension2DataTypeStr=Inherit: Inherit from 'Breakpoint data'  Table=mTmComprCtrl_n_u16FFBattCooltRpmChargingNhp  TableDataTypeStr=Inherit: Inherit from 'Table data'  ExtrapMethod=Clip  InternalRulePriority=Speed  OutDataTypeStr=Inherit: Inherit via back propagation  RndMeth=Simplest  InputSameDT=off
      settings: InputPortMap=u0,u1
  2-D Lookup Table3 : Lookup_n-D  LookupTableObject=mTmComprCtrl_n_u16FFBattCooltRpmCharging  BreakpointsForDimension1=mTmComprCtrl_n_u16FFBattCooltRpmCharging_Y  BreakpointsForDimension2=mTmComprCtrl_n_u16FFBattCooltRpmCharging_X  BreakpointsForDimension1DataTypeStr=Inherit: Inherit from 'Breakpoint data'  BreakpointsForDimension2DataTypeStr=Inherit: Inherit from 'Breakpoint data'  Table=mTmComprCtrl_n_u16FFBattCooltRpmCharging  TableDataTypeStr=Inherit: Inherit from 'Table data'  ExtrapMethod=Clip  InternalRulePriority=Speed  OutDataTypeStr=Inherit: Inherit via back propagation  RndMeth=Simplest  InputSameDT=off
      settings: InputPortMap=u0,u1
  2-D Lookup Table4 : Lookup_n-D  LookupTableObject=mTmComprCtrl_n_u16FFBattCooltRpmCharging  BreakpointsForDimension1=mTmComprCtrl_n_u16FFBattCooltRpmSuperCharging_Y  BreakpointsForDimension2=mTmComprCtrl_n_u16FFBattCooltRpmSuperCharging_X  BreakpointsForDimension1DataTypeStr=Inherit: Inherit from 'Breakpoint data'  BreakpointsForDimension2DataTypeStr=Inherit: Inherit from 'Breakpoint data'  Table=mTmComprCtrl_n_u16FFBattCooltRpmSuperCharging  TableDataTypeStr=Inherit: Inherit from 'Table data'  ExtrapMethod=Clip  InternalRulePriority=Speed  OutDataTypeStr=Inherit: Inherit via back propagation  RndMeth=Simplest  InputSameDT=off
      settings: InputPortMap=u0,u1
  2-D Lookup Table5 : Lookup_n-D  LookupTableObject=mTmComprCtrl_n_u16FFBattCooltRpmCharging  BreakpointsForDimension1=mTmComprCtrl_n_u16FFBattCooltRpmSuperChargingNhp_Y  BreakpointsForDimension2=mTmComprCtrl_n_u16FFBattCooltRpmSuperChargingNhp_X  BreakpointsForDimension1DataTypeStr=Inherit: Inherit from 'Breakpoint data'  BreakpointsForDimension2DataTypeStr=Inherit: Inherit from 'Breakpoint data'  Table=mTmComprCtrl_n_u16FFBattCooltRpmSuperChargingNhp  TableDataTypeStr=Inherit: Inherit from 'Table data'  ExtrapMethod=Clip  InternalRulePriority=Speed  OutDataTypeStr=Inherit: Inherit via back propagation  RndMeth=Simplest  InputSameDT=off
      settings: InputPortMap=u0,u1
  Compare To Constant : simulink/Logic and Bit Operations/Compare To Constant  relop===  const=2  OutDataTypeStr=boolean
  Multiport Switch : MultiPortSwitch  DataPortOrder=Specify indices  DataPortIndices={2,12}  DataPortForDefault=Additional data port  DiagnosticForDefault=None  SaturateOnIntegerOverflow=off  InputSameDT=off
  Multiport Switch1 : MultiPortSwitch  DataPortOrder=Specify indices  DataPortIndices={2,12}  DataPortForDefault=Additional data port  DiagnosticForDefault=None  SaturateOnIntegerOverflow=off  InputSameDT=off
  Product : Product  OutDataTypeStr=uint16
  Switch : Switch  Criteria=u2 ~= 0  SaturateOnIntegerOverflow=off  InputSameDT=off
  SM1FF : Outport
  wires:
  2-D Lookup Table4/1 -> Multiport Switch/4
  2-D Lookup Table3/1 -> Multiport Switch/3
  [sTmIn_D_u8DCChrgSt] -> Multiport Switch/1
  2-D Lookup Table/1 -> Multiport Switch/2
  [sTmSigProces_D_u8HvBattCoolgReq] -> 2-D Lookup Table4/1, 2-D Lookup Table3/1, 2-D Lookup Table/1
  [sTmIn_Te_s32HvBattCooltTReq] -> 2-D Lookup Table3/2, 2-D Lookup Table4/2, 2-D Lookup Table/2
  sTmIn_Te_s32HvBattCooltTReq/1 -> [sTmIn_Te_s32HvBattCooltTReq]
  sTmIn_D_u8DCChrgSt/1 -> [sTmIn_D_u8DCChrgSt]
  sTmSigProces_D_u8HvBattCoolgReq/1 -> [sTmSigProces_D_u8HvBattCoolgReq]
  [sTmSigProces_Te_s32TAmb] -> 1-D Lookup Table/1
  Switch/1 -> Product/1  "rTmComprCtrl_fac_s32SM1FFRaw"
  1-D Lookup Table/1 -> Product/2  "rTmComprCtrl_fac_s32SM1FFTFactor"
  Product/1 -> SM1FF/1  "SM1FF"
  sTmSigProces_Te_s32TAmb/1 -> [sTmSigProces_Te_s32TAmb]
  2-D Lookup Table5/1 -> Multiport Switch1/4
  2-D Lookup Table1/1 -> Multiport Switch1/2
  [sTmIn_D_u8DCChrgSt] -> Multiport Switch1/1
  2-D Lookup Table2/1 -> Multiport Switch1/3
  [sTmSigProces_D_u8HvBattCoolgReq] -> 2-D Lookup Table5/1, 2-D Lookup Table2/1, 2-D Lookup Table1/1
  [sTmIn_Te_s32HvBattCooltTReq] -> 2-D Lookup Table5/2, 2-D Lookup Table2/2, 2-D Lookup Table1/2
  Compare To Constant/1 -> Switch/2
  [sTmIn_D_u8HeatPump] -> Compare To Constant/1
  Multiport Switch/1 -> Switch/1
  Multiport Switch1/1 -> Switch/3
  sTmIn_D_u8HeatPump/1 -> [sTmIn_D_u8HeatPump]

== system ScriptDemo/Create/createMerge/Before/SM1SM21/ID26247_SM1Error ==
  sTmIn_Te_s32HvBattCooltTReq : Inport
  sTmSigProces_Te_s32HvBattCooltTFilter : Inport  Port=2
  "NegAndPosCheck " : Subsystem  AncestorBlock=CustomLib/TempNegAndPosCheck
  Saturation : Saturate  UpperLimit=40  LowerLimit=12
  Terminator : Terminator
  rTmComprCtrl_Te_s32TempError : Outport  OutDataTypeStr=single
  wires:
  sTmSigProces_Te_s32HvBattCooltTFilter/1 -> "NegAndPosCheck "/2(Acture)
  sTmIn_Te_s32HvBattCooltTReq/1 -> Saturation/1
  "NegAndPosCheck "/2(Dvt_PosFlag) -> Terminator/1
  Saturation/1 -> "NegAndPosCheck "/1(SetPoint)
  "NegAndPosCheck "/1(Dvt) -> rTmComprCtrl_Te_s32TempError/1

== system ScriptDemo/Create/createMerge/Before/SM1SM21/SM1FFEnable ==
  xTmComprCtrl_B_CompOnReqCompOn : Inport  OutDataTypeStr=boolean
  BevvFFPeriod : Subsystem  mask{CounterLim=cTmComprCtrl_t_u16BattCooltFFPeriod}
      mask DialogControl ParameterGroupVar Prompt: 参数
  Compare To Constant2 : simulink/Logic and Bit Operations/Compare To Constant  relop===  const=0  OutDataTypeStr=boolean
  Compare To Constant3 : simulink/Logic and Bit Operations/Compare To Constant  relop===  const=1  OutDataTypeStr=boolean
  Logical Operator3 : Logic  AllPortsSameDT=off  OutDataTypeStr=boolean
  Unit Delay : UnitDelay  SampleTime=-1  HasFrameUpgradeWarning=on
  SM1FFEnable_B_SM1FFEnable : Outport  OutDataTypeStr=boolean
  wires:
  Unit Delay/1 -> Compare To Constant2/1
  [xTmComprCtrl_B_CompOnReqCompOn] -> Compare To Constant3/1, Unit Delay/1
  Compare To Constant2/1 -> Logical Operator3/1
  Logical Operator3/1 -> BevvFFPeriod/1(Counter_Reset)
  Compare To Constant3/1 -> Logical Operator3/2
  BevvFFPeriod/1(Counter_Trig) -> SM1FFEnable_B_SM1FFEnable/1
  xTmComprCtrl_B_CompOnReqCompOn/1 -> [xTmComprCtrl_B_CompOnReqCompOn]

== system ScriptDemo/Create/createMerge/Before/SM1SM21/SM1_Ki ==
  sTmSigProces_D_u8BattThermReq : Inport
  sTmIn_D_u8DCChrgSt : Inport  Port=2
  sTmSigProces_D_u8HvBattCoolgReq : Inport  Port=3
  rTmComprCtrl_Te_s32TempError : Inport  Port=4
  2-D Lookup Table10 : Lookup_n-D  LookupTableObject=mTmComprCtrl_n_u16FFBattCooltRpmCharging  BreakpointsForDimension1=mTmComprCtrl_n_u16KiBattCooltRpmSuperCharging_Y  BreakpointsForDimension2=mTmComprCtrl_n_u16KiBattCooltRpmSuperCharging_X  BreakpointsForDimension1DataTypeStr=Inherit: Inherit from 'Breakpoint data'  BreakpointsForDimension2DataTypeStr=Inherit: Inherit from 'Breakpoint data'  Table=mTmComprCtrl_n_u16KiBattCooltRpmSuperCharging  TableDataTypeStr=Inherit: Inherit from 'Table data'  ExtrapMethod=Clip  InternalRulePriority=Speed  OutDataTypeStr=Inherit: Inherit via back propagation  RndMeth=Simplest  InputSameDT=off
      settings: InputPortMap=u0,u1
  2-D Lookup Table8 : Lookup_n-D  LookupTableObject=mTmComprCtrl_n_u16FFBattCooltRpmCharging  BreakpointsForDimension1=mTmComprCtrl_n_u16KiBattCooltRpmNorm_Y  BreakpointsForDimension2=mTmComprCtrl_n_u16KiBattCooltRpmNorm_X  BreakpointsForDimension1DataTypeStr=Inherit: Inherit from 'Breakpoint data'  BreakpointsForDimension2DataTypeStr=Inherit: Inherit from 'Breakpoint data'  Table=mTmComprCtrl_n_u16KiBattCooltRpmNorm  TableDataTypeStr=Inherit: Inherit from 'Table data'  ExtrapMethod=Clip  InternalRulePriority=Speed  OutDataTypeStr=Inherit: Inherit via back propagation  RndMeth=Simplest  InputSameDT=off
      settings: InputPortMap=u0,u1
  2-D Lookup Table9 : Lookup_n-D  LookupTableObject=mTmComprCtrl_n_u16FFBattCooltRpmCharging  BreakpointsForDimension1=mTmComprCtrl_n_u16KiBattCooltRpmCharging_Y  BreakpointsForDimension2=mTmComprCtrl_n_u16KiBattCooltRpmCharging_X  BreakpointsForDimension1DataTypeStr=Inherit: Inherit from 'Breakpoint data'  BreakpointsForDimension2DataTypeStr=Inherit: Inherit from 'Breakpoint data'  Table=mTmComprCtrl_n_u16KiBattCooltRpmCharging  TableDataTypeStr=Inherit: Inherit from 'Table data'  ExtrapMethod=Clip  InternalRulePriority=Speed  OutDataTypeStr=Inherit: Inherit via back propagation  RndMeth=Simplest  InputSameDT=off
      settings: InputPortMap=u0,u1
  tableChoose : Subsystem
  SM1Ki : Outport
  wires:
  sTmIn_D_u8DCChrgSt/1 -> tableChoose/2(sTmIn_D_u8DCChrgSt)
  sTmSigProces_D_u8BattThermReq/1 -> tableChoose/1(sTmSigProces_D_u8BattThermReq)
  2-D Lookup Table10/1 -> tableChoose/5(tab3)
  2-D Lookup Table8/1 -> tableChoose/3(tab1)
  2-D Lookup Table9/1 -> tableChoose/4(tab2)
  sTmSigProces_D_u8HvBattCoolgReq/1 -> 2-D Lookup Table8/1, 2-D Lookup Table10/1, 2-D Lookup Table9/1
  rTmComprCtrl_Te_s32TempError/1 -> 2-D Lookup Table8/2, 2-D Lookup Table10/2, 2-D Lookup Table9/2
  tableChoose/1(out) -> SM1Ki/1
